simulink model "autopilota_v_22_last"  (R2020b)
settings: Solver=ode4  StartTime=0.0  StopTime=300  FixedStep=0.02  RelTol=1e-3
values from neighbouring files (symbols this model uses):
  alphavec_rad = deg2rad(alphavec)    [v2021_10_27_calcoloAerodinamica.m]
  attuatore_Amax = 20*(pi/180)    (= 0.349065850399)    [v2021_10_27_avvioSITL.m]    (also in v2021_10_27_calcoloAerodinamica.m)
  attuatore_Amin = -20*(pi/180)    (= -0.349065850399)    [v2021_10_27_avvioSITL.m]
  attuatore_Emax = 25*(pi/180)    (= 0.436332312999)    [v2021_10_27_avvioSITL.m]    (also in v2021_10_27_calcoloAerodinamica.m)
  attuatore_Emin = -25*(pi/180)    (= -0.436332312999)    [v2021_10_27_avvioSITL.m]
  attuatore_Rmax = 25*(pi/180)    (= 0.436332312999)    [v2021_10_27_avvioSITL.m]    (also in v2021_10_27_calcoloAerodinamica.m)
  attuatore_Rmin = -25*(pi/180)    (= -0.436332312999)    [v2021_10_27_avvioSITL.m]
  attuatore_Tmax = 0.99    [v2021_10_27_avvioSITL.m]
  attuatore_Tmin = 0    [v2021_10_27_avvioSITL.m]
  b = 2.62    [v2021_10_27_calcoloAerodinamica.m]
  betavec_rad = deg2rad(betavec)    [v2021_10_27_calcoloAerodinamica.m]
  bias = [baccxINI,baccyINI,bacczINI,bpINI,bqINI,brINI]    [v2021_10_27_avvioSITL.m]
  c = .32    (= 0.32)    [v2021_10_27_calcoloAerodinamica.m]
  cbar = .32    (= 0.32)    [v2021_10_27_calcoloAerodinamica.m]
  CD0 = 0.024    [v2021_10_27_calcoloAerodinamica.m]
  Clp = -0.5058    [v2021_10_27_calcoloAerodinamica.m]
  CLq = 19.166    [v2021_10_27_calcoloAerodinamica.m]
  Clr = 0.1459    [v2021_10_27_calcoloAerodinamica.m]
  Cmq = -81.796    [v2021_10_27_calcoloAerodinamica.m]
  Cnp = 0.007507    [v2021_10_27_calcoloAerodinamica.m]
  Cnr = -1.2593    [v2021_10_27_calcoloAerodinamica.m]
  CYp = 0.050728    [v2021_10_27_calcoloAerodinamica.m]
  CYr = 0.358925    [v2021_10_27_calcoloAerodinamica.m]
  deltaTtrim = 0.1    [v2021_10_27_avvioSITL.m]
  Dprop = 2*Rprop    (= 0.5334)    [v2021_10_27_calcoloAerodinamica.m]
  final_h = 35    [v2021_10_27_avvioSITL.m]
  g = [0 0 9.81]'    [v2021_10_27_calcoloAerodinamica.m]
  HINI = -State0.Pos0(3)    [v2021_10_27_avvioSITL.m]
  interventoA_05 = 20*0.8    (= 16)    [v2021_10_27_avvioSITL.m]
  interventoA_1 = 10    [v2021_10_27_avvioSITL.m]
  interventoE_05 = 25*0.8    (= 20)    [v2021_10_27_avvioSITL.m]
  interventoE_1 = 10    [v2021_10_27_avvioSITL.m]
  interventoT = 1*0.6    (= 0.6)    [v2021_10_27_avvioSITL.m]
  inv_A = 1    [v2021_10_27_avvioSITL.m]
  inv_comp_h = 1    [v2021_10_27_avvioSITL.m]
  inv_E = 1    [v2021_10_27_avvioSITL.m]
  inv_R = 1    [v2021_10_27_avvioSITL.m]
  inv_T = 1    [v2021_10_27_avvioSITL.m]
  Jeng = 0    [v2021_10_27_calcoloAerodinamica.m]
  Jprop = mprop*(Dprop^2)/12    (= 0.00422031414)    [v2021_10_27_calcoloAerodinamica.m]
  K_AW_B_AP_quota = 1000    [v2021_10_27_avvioSITL.m]
  K_AW_B_becc = -250    [v2021_10_27_avvioSITL.m]
  K_AW_B_imb = 0    [v2021_10_27_avvioSITL.m]
  K_AW_B_roll = 500    [v2021_10_27_avvioSITL.m]
  K_imb_inv = -0.001306    [v2021_10_27_avvioSITL.m]
  Kd_AP_rotta = 0.995    [v2021_10_27_avvioSITL.m]
  Kd_h_app = 0.085    [v2021_10_27_avvioSITL.m]
  Kd_h_flare = 0.01    [v2021_10_27_avvioSITL.m]
  Ki_AP_quota_select = 0.01936    [v2021_10_27_avvioSITL.m]
  Ki_AP_rotta = 0.002    [v2021_10_27_avvioSITL.m]
  Ki_AP_vel = 0.025175    [v2021_10_27_avvioSITL.m]
  Ki_becch = -0.1963    [v2021_10_27_avvioSITL.m]
  Ki_h_app = 0.055    [v2021_10_27_avvioSITL.m]
  Ki_h_cruise = 0.008    [v2021_10_27_avvioSITL.m]
  Ki_h_flare = 0.07    [v2021_10_27_avvioSITL.m]
  Ki_roll = 0.004528    [v2021_10_27_avvioSITL.m]
  Kp_AP_quota_hold_h = 0.5503    [v2021_10_27_avvioSITL.m]
  Kp_AP_quota_hold_l = 0.5503    [v2021_10_27_avvioSITL.m]
  Kp_AP_quota_select = 0.02647    [v2021_10_27_avvioSITL.m]
  Kp_AP_rotta = 0.520    (= 0.52)    [v2021_10_27_avvioSITL.m]
  Kp_AP_vel = 0.132175    [v2021_10_27_avvioSITL.m]
  Kp_becch = -0.30    (= -0.3)    [v2021_10_27_avvioSITL.m]
  Kp_comp_h = 0.035    [v2021_10_27_avvioSITL.m]
  Kp_h_app_max = 0.086    [v2021_10_27_avvioSITL.m]
  Kp_h_app_min = 0.01    [v2021_10_27_avvioSITL.m]
  Kp_h_cruise = 0.04    [v2021_10_27_avvioSITL.m]
  Kp_h_flare = 0.1    [v2021_10_27_avvioSITL.m]
  Kp_imb = 0.0019415    [v2021_10_27_avvioSITL.m]
  Kp_p = 0.006913    [v2021_10_27_avvioSITL.m]
  Kp_q = -0.025    [v2021_10_27_avvioSITL.m]
  Kp_roll = 0.0718    [v2021_10_27_avvioSITL.m]
  Kp_Rotta_ATO = 4    [v2021_10_27_avvioSITL.m]
  Kp_Rotta_psi = -0.01    [v2021_10_27_avvioSITL.m]
  latitudineINI = 41.854432*pi/180    (= 0.730497644952)    [v2021_10_27_avvioSITL.m]
  longitudineINI = 12.306650*pi/180    (= 0.214791562391)    [v2021_10_27_avvioSITL.m]
  matricepolinomi = [0.0816560564319 0.0869820125665 0.0279748858868 -4.51852057237 0.0146653626785 -0.925775006168 8.18052218957e-06 -1.47322908992e-05 7.59644694438e-06 0.00246695371279 9.02269223066e-06 0.000559334242525 ... (126 elements, 6x21)]    [coefficienti_curve_renard.mat]
  q = stato(11)    [measure_F1B.m]
  Q1B = [    2e-15;     2e-15 ... (first row only)    [COV_F1B.m]
  r = stato(12)    [measure_F1B.m]
  R1B = [     2e-14;             2e-14 ... (first row only)    [COV_F1B.m]
  rACtG = rACtP-rGP    [v2021_10_27_calcoloAerodinamica.m]
  rACwG = rACwP-rGP    [v2021_10_27_calcoloAerodinamica.m]
  rAHRSG = rAHRSP-rGP    [v2021_10_27_calcoloAerodinamica.m]
  rho = 1.21330    (= 1.2133)    [v2021_10_27_calcoloAerodinamica.m]
  rLEG = rLEP-rGP    [v2021_10_27_calcoloAerodinamica.m]
  rmglG = rmglP-rGP    [v2021_10_27_calcoloAerodinamica.m]
  rmgrG = rmgrP-rGP    [v2021_10_27_calcoloAerodinamica.m]
  rngG = rngP-rGP    [v2021_10_27_calcoloAerodinamica.m]
  rNPG = rNPP-rGP    [v2021_10_27_calcoloAerodinamica.m]
  rPG = -rGP    [v2021_10_27_calcoloAerodinamica.m]
  Rprop = 0.2667    [v2021_10_27_calcoloAerodinamica.m]
  S = b*cbar    (= 0.8384)    [v2021_10_27_calcoloAerodinamica.m]
  safe_phi = 55    [v2021_10_27_avvioSITL.m]
  safe_V = 40    [v2021_10_27_avvioSITL.m]
  Sensor_Offsets = [0,0,0]    [v2021_10_27_avvioSITL.m]
  T_cal = 0.4    [v2021_10_27_avvioSITL.m]
  theta_rot = 10    [v2021_10_27_avvioSITL.m]
  time_alarm_SAFE = 300    [v2021_10_27_avvioSITL.m]
  tsamp = 0.02    [v2021_10_27_avvioSITL.m]
  update = [2,2,2]    [v2021_10_27_avvioSITL.m]
  V_max = 35    [v2021_10_27_avvioSITL.m]
  V_stall = 15    [v2021_10_27_avvioSITL.m]
  vd_ini = 0    [v2021_10_27_avvioSITL.m]
  vel_wp1_al = 25    [v2021_10_27_avvioSITL.m]
  vel_wp2_al = 20    [v2021_10_27_avvioSITL.m]
  W = m*g    [v2021_10_27_calcoloAerodinamica.m]
  Zeng = rPG(3)    [v2021_10_27_calcoloAerodinamica.m]
undefined symbols (not defined in the file or in its folder): CldA, CLdE, CldR, CmdE, CndA, CndR, CYdA, CYdR, DiscIntNeverNeededParam, Earth, F, J_vec, MIL, Newton, Raphson, t_AP, WGS84
libraries: simulink_extras x38, pid_lib x9, simulink x5, dspsigops x4, aerolibwind2 x3, aerolibasang x2, aerolibtransform2sys x2, aerolibtransform2 x2, aerosimlib x1, shared6dof x1, aerolibatmos2 x1
(part 4 of 12)

== system autopilota_v_22_last/Subsystem1/Subsystem1/Subsystem ==
  modo : Inport
  rotta : Inport  Port=2
  velocita : Inport  Port=3
  quota : Inport  Port=4
  RC : Inport  Port=5
  heading : Inport  Port=6
  TAS : Inport  Port=7
  h : Inport  Port=8
  RC_default : Inport  Port=9
  <IAS> : Inport  Port=10
  <ALT> : Inport  Port=11
  <HDG> : Inport  Port=12
  <RC> : Inport  Port=13
  <Ingaggio_AP> : Inport  Port=14
  Enable : EnablePort
  Abs : Abs
  Data Type Conversion{,1..3} (4 alike) : DataTypeConversion  OutDataTypeStr=double
  Memory{,1..3,6} (5 alike) : Memory  InheritSampleTime=on
  Radians to Degrees3 : simulink_extras/Transformations/Radians to Degrees
  VETTORIALE : MATLAB Function  TreatAsAtomicUnit=on
  Out1 : Outport  VectorParamsAs1DForOutWhenUnconnected=off
  Out2 : Outport  Port=2  VectorParamsAs1DForOutWhenUnconnected=off
  Out3 : Outport  Port=3  VectorParamsAs1DForOutWhenUnconnected=off
  Out4 : Outport  Port=4  VectorParamsAs1DForOutWhenUnconnected=off
  wires:
  Data Type Conversion1/1 -> VETTORIALE/8(VELOCITA)
  Memory1/1 -> VETTORIALE/18(ALT_pre)
  VETTORIALE/5(ingaggio_AP_mem) -> Memory6/1
  Data Type Conversion2/1 -> VETTORIALE/9(QUOTA)
  VETTORIALE/8(ALT_pre_mem) -> Memory1/1
  Radians to Degrees3/1 -> VETTORIALE/11(HEADING)
  Memory6/1 -> VETTORIALE/15(ingaggio_AP_pre)
  h/1 -> VETTORIALE/13(h)
  Memory3/1 -> VETTORIALE/16(modo_pre)
  VETTORIALE/6(modo_pre_mem) -> Memory3/1
  Abs/1 -> VETTORIALE/10(RC)
  VETTORIALE/9(HDG_pre_mem) -> Memory/1
  Data Type Conversion3/1 -> Abs/1
  Memory/1 -> VETTORIALE/19(HDG_pre)
  Data Type Conversion/1 -> VETTORIALE/7(ROTTA)
  Memory2/1 -> VETTORIALE/17(IAS_pre)
  VETTORIALE/7(IAS_pre_mem) -> Memory2/1
  VETTORIALE/3(rotta_vett) -> Out3/1
  modo/1 -> VETTORIALE/1(modo)
  <ALT>/1 -> VETTORIALE/3(ALT)
  <RC>/1 -> VETTORIALE/5(I_RC)
  RC/1 -> Data Type Conversion3/1
  quota/1 -> Data Type Conversion2/1
  <Ingaggio_AP>/1 -> VETTORIALE/6(ingaggio_AP)
  TAS/1 -> VETTORIALE/12(TAS)
  heading/1 -> Radians to Degrees3/1
  velocita/1 -> Data Type Conversion1/1
  VETTORIALE/1(V_vett) -> Out1/1
  VETTORIALE/2(h_vett) -> Out2/1
  <IAS>/1 -> VETTORIALE/2(IAS)
  rotta/1 -> Data Type Conversion/1
  RC_default/1 -> VETTORIALE/14(RC_default)
  VETTORIALE/4(RC_vett) -> Out4/1
  <HDG>/1 -> VETTORIALE/4(HDG)

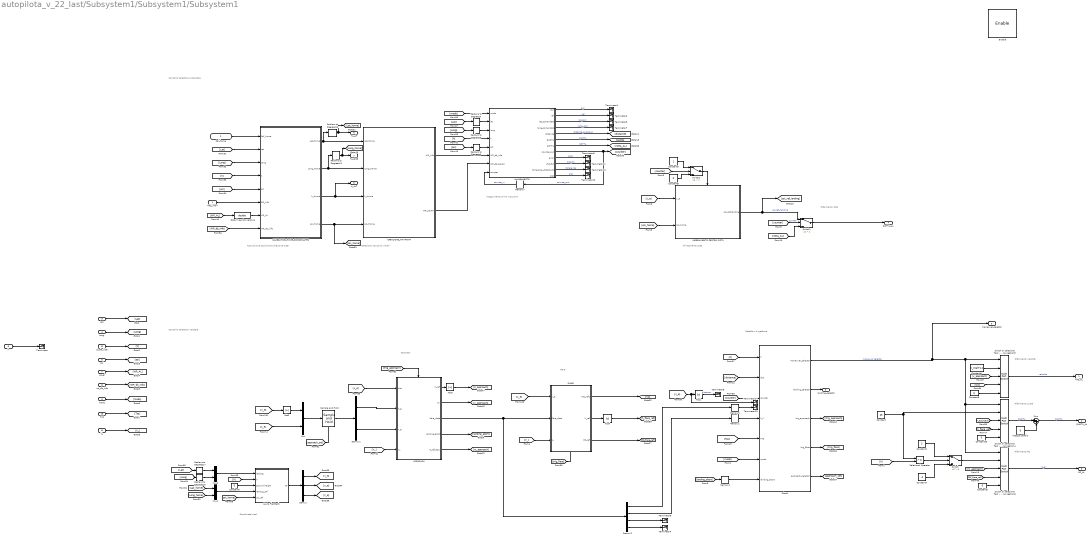
== system autopilota_v_22_last/Subsystem1/Subsystem1/Subsystem1 ==
  note: Approach
  note: Controllo traiettoria verticale
  note: Flare
  note: Coordinate locali
  note: Stateflow di gestione
  note: Controllo traiettoria orizzontale
  note: Acquisizione posizione
      | e direzione pista
  note: Creazione waypoint
      | virtuali
  note: Inseguimento primo
      | waypoint
  note: Allineamento
      | pista
  note: Riferimento rotta
  note: Riferimento velocità
  note: Riferimento quota
  note: Riferimento RC
  <GC_info> : Inport
  Cal_home : Inport  Port=2
  Lat : Inport  Port=3
  Long : Inport  Port=4
  h : Inport  Port=5
  psi : Inport  Port=6
  wp_al : Inport  Port=7
  wp_db_info : Inport  Port=8
  modo : Inport  Port=9
  TAS : Inport  Port=10
  V_ : Inport  Port=11
  quota_lidar : Inport  Port=12
  Enable : EnablePort
  ALLINEAMENTO : MATLAB Function  TreatAsAtomicUnit=on
  APPROACH : Subsystem
  Abs{1..4} (4 alike) : Abs
  CALIBRATING_HOME_COORDINATES : MATLAB Function  TreatAsAtomicUnit=on
  "CREAZIONE_WAYPOINT " : Subsystem
  Chart1 : Stateflow chart  TreatAsAtomicUnit=on
  Constant : Constant  Value=45
  Constant1 : Constant  Value=2  SampleTime=0.02
  Constant{5,8..10} (4 alike) : Constant  Value=0
  Constant3 : Constant
  Constant4 : Constant  Value=0  SampleTime=0.02
  Constant6 : Constant  Value=V_stall*1.4  SampleTime=0.02
  Constant7 : Constant  Value=-2  SampleTime=0.02
  Data Type Conversion4 : DataTypeConversion  OutDataTypeStr=double
  Demux : Demux  Outputs=3
  Demux1 : Demux  Outputs=2
  Demux2 : Demux
  FLARE : Subsystem
  INSEGUIMENTO CENTRO PISTA : Subsystem
  LLA to Flat Earth : Subsystem
  Memory1 : Memory
  Memory2 : Memory
  Memory5 : Memory
  Memory7 : Memory  InitialCondition=1  InheritSampleTime=on
  Mux : Mux  Inputs=2
  Mux1 : Mux  Inputs=2
  Mux2 : Mux  Inputs=2
  Radians to Degrees{4..6,10..11,16..17} (7 alike) : simulink_extras/Transformations/Radians to Degrees
  Relational Operator : RelationalOperator  OutDataTypeStr=boolean  RndMeth=Simplest
  Sample and Hold : dspsigops/Sample and Hold  trig=Rising edge  initCond=[0 0]  latchinput=off
  Sum : Sum  Inputs=|++
  Switch : Switch  Criteria=u2 > Threshold
  Switch di selezione Task - Waypoint navigation4 : MultiPortSwitch  Inputs=4
  Switch di selezione Task - Waypoint navigation5 : MultiPortSwitch  Inputs=4
  Switch di selezione Task - Waypoint navigation6 : MultiPortSwitch  Inputs=4
  Switch1 : Switch  Criteria=u2 > Threshold  Threshold=1
  Switch2 : Switch  Criteria=u2 > Threshold  Threshold=1
  Terminator{,1..5,7..14} (14 alike) : Terminator
  latezza carrello : Constant  Value=0
  TAS_AL : Outport  VectorParamsAs1DForOutWhenUnconnected=off
  QUOTA_AL : Outport  Port=2  VectorParamsAs1DForOutWhenUnconnected=off
  RC_AL : Outport  Port=3  VectorParamsAs1DForOutWhenUnconnected=off
  ROTTA_AL : Outport  Port=4  VectorParamsAs1DForOutWhenUnconnected=off
  landing_selector : Outport  Port=5  VectorParamsAs1DForOutWhenUnconnected=off
  H_LAT : Outport  Port=6  VectorParamsAs1DForOutWhenUnconnected=off
  H_LONG : Outport  Port=7  VectorParamsAs1DForOutWhenUnconnected=off
  H_ALT : Outport  Port=8  VectorParamsAs1DForOutWhenUnconnected=off
  maneuver_selector : Outport  Port=9
  wires:
  Chart1/1(maneuver_selector) -> maneuver_selector/1, Switch di selezione Task - Waypoint navigation6/1, Switch di selezione Task - Waypoint navigation4/1, Switch di selezione Task - Waypoint navigation5/1  "maneuver selector"
  LLA to Flat Earth/1(Xe) -> Demux/1
  Radians to Degrees11/1 -> H_LONG/1, [Long_home]
  Mux/1 -> Sample and Hold/1
  ALLINEAMENTO/4(long_comandato) -> Terminator7/1  "long_com"
  Mux1/1 -> LLA to Flat Earth/4(latlong_ref)
  [WP_db_info] -> CALIBRATING_HOME_COORDINATES/8(WP_db_info)
  Demux1/2 -> APPROACH/3(x_g)
  Abs2/1 -> Mux/1
  ALLINEAMENTO/3(lat_comandato) -> Terminator5/1  "lat_com"
  [rc_approach] -> Switch di selezione Task - Waypoint navigation6/3
  [V2] -> Switch di selezione Task - Waypoint navigation5/4
  [x_e] -> Terminator14/1, Abs1/1
  Abs4/1 -> [h_flare_ref]
  CALIBRATING_HOME_COORDINATES/3(h_Home) -> H_ALT/1, "CREAZIONE_WAYPOINT "/3(h_Home)
  [h] -> Chart1/1(h)
  [x_e] -> FLARE/1(x_e)
  [Long_home] -> Mux1/2
  APPROACH/3(flare_data) -> Demux2/1, FLARE/2(flare_data)
  CALIBRATING_HOME_COORDINATES/1(Lat_Home) -> Radians to Degrees10/1, "CREAZIONE_WAYPOINT "/1(Lat_Home)
  Demux/2 -> [y_e]
  FLARE/3(RC_ref) -> [RC_flare_ref]
  Chart1/4(trig_flare) -> [trig_flare]
  [h] -> LLA to Flat Earth/2(h)
  [Long] -> Radians to Degrees16/1
  Demux/3 -> [z_e]
  Demux2/2 -> Memory1/1
  Radians to Degrees10/1 -> H_LAT/1, [Lat_home]
  Sample and Hold/1 -> Demux1/1
  [trig_approach] -> APPROACH/Enable
  Switch/1 -> Switch di selezione Task - Waypoint navigation6/2
  Memory5/1 -> Terminator13/1
  Cal_home/1 -> CALIBRATING_HOME_COORDINATES/1(Cal_home)
  Demux2/3 -> Terminator3/1
  FLARE/2(h_ref) -> Abs4/1
  [z_e] -> Abs2/1
  [x_e] -> Mux/2
  CALIBRATING_HOME_COORDINATES/2(Long_Home) -> "CREAZIONE_WAYPOINT "/2(Long_Home), Radians to Degrees11/1
  Demux2/4 -> Terminator4/1
  FLARE/1(Tas_ref1) -> [V2]
  ALLINEAMENTO/7(ROTTA) -> [rotta_AL]  "ROTTA"
  APPROACH/2(V1) -> [v_approach]
  [V_] -> FLARE/3(V_)
  Chart1/5(approach_selector) -> [approach_sel]
  [h_approach] -> Switch di selezione Task - Waypoint navigation4/3
  [RC_flare_ref] -> Switch di selezione Task - Waypoint navigation6/4
  Chart1/3(trig_approach) -> [trig_approach]
  [Lat_home] -> Mux1/1
  ALLINEAMENTO/6(QUOTA) -> [quota]  "QUOTA"
  ALLINEAMENTO/8(counter_out) -> Memory7/1, [counter]  "counter_out"
  Demux/1 -> [x_e]
  Demux2/1 -> Memory5/1
  CALIBRATING_HOME_COORDINATES/4(psi_Home) -> [psi_home], "CREAZIONE_WAYPOINT "/4(psi_Home)
  Abs3/1 -> [h_approach]
  Mux2/1 -> LLA to Flat Earth/1(latlong)
  Chart1/2(landing_selector) -> landing_selector/1
  Constant/1 -> Switch di selezione Task - Waypoint navigation4/2, Relational Operator/1
  [h_flare_ref] -> Switch di selezione Task - Waypoint navigation4/4
  [v_approach] -> Switch di selezione Task - Waypoint navigation5/3
  [Tas] -> Chart1/5(TAS)
  APPROACH/1(h_ref) -> Abs3/1
  Data Type Conversion4/1 -> CALIBRATING_HOME_COORDINATES/7(WP_AL)
  [Lat] -> Radians to Degrees17/1
  Demux1/1 -> APPROACH/2(h_g)
  Constant4/1 -> LLA to Flat Earth/3(ground height)
  [psi] -> CALIBRATING_HOME_COORDINATES/5(psi)
  ALLINEAMENTO/2(vel) -> Terminator2/1  "vel"
  Radians to Degrees5/1 -> ALLINEAMENTO/3(long)
  [x_e] -> APPROACH/1(dist)
  Memory7/1 -> ALLINEAMENTO/8(counter)  "counter_in"
  [h] -> CALIBRATING_HOME_COORDINATES/4(h)
  [counter] -> Chart1/3(counter)
  Radians to Degrees4/1 -> ALLINEAMENTO/2(lat)
  [approach_sel] -> Sample and Hold/Trigger
  [Lat] -> Radians to Degrees4/1
  "CREAZIONE_WAYPOINT "/2(WP_param) -> ALLINEAMENTO/7(WP_db_param)
  [h] -> ALLINEAMENTO/4(h)
  [Long] -> Radians to Degrees5/1
  <GC_info>/1 -> CALIBRATING_HOME_COORDINATES/6(GC_info)
  ALLINEAMENTO/1(e_h) -> Terminator1/1  "e_h"
  Radians to Degrees6/1 -> ALLINEAMENTO/5(psi)
  Radians to Degrees16/1 -> Mux2/2
  [psi] -> Radians to Degrees6/1
  [WP_AL] -> Data Type Conversion4/1
  [modo] -> ALLINEAMENTO/1(modo)
  ALLINEAMENTO/5(distance) -> [distance]  "distance_autoland"
  Radians to Degrees17/1 -> Mux2/1
  "CREAZIONE_WAYPOINT "/1(WP_info) -> ALLINEAMENTO/6(WP_db_info)
  [trig_flare] -> FLARE/Enable
  Constant6/1 -> Switch di selezione Task - Waypoint navigation5/2
  [psi_home] -> LLA to Flat Earth/5(psi_ref)
  Sum/1 -> QUOTA_AL/1  "QUOTA"
  Switch di selezione Task - Waypoint navigation6/1 -> RC_AL/1  "rc_al"
  Switch di selezione Task - Waypoint navigation5/1 -> TAS_AL/1  "velocita"
  Lat/1 -> [Lat]
  Long/1 -> [Long]
  h/1 -> Terminator/1
  psi/1 -> [psi]
  wp_al/1 -> [WP_AL]
  wp_db_info/1 -> [WP_db_info]
  modo/1 -> [modo]
  TAS/1 -> [Tas]
  V_/1 -> [V_]
  Switch1/1 -> ROTTA_AL/1
  [h] -> Relational Operator/2
  Relational Operator/1 -> Switch/2
  Constant1/1 -> Switch/1
  Constant7/1 -> Switch/3
  [modo] -> Chart1/6(modo)
  APPROACH/4(landing_abort) -> [landing_abort]
  Memory1/1 -> Chart1/4(h_f)
  Memory2/1 -> Chart1/7(landing_abort)
  [landing_abort] -> Memory2/1
  [Lat] -> CALIBRATING_HOME_COORDINATES/2(Lat)
  [Long] -> CALIBRATING_HOME_COORDINATES/3(Long)
  [counter] -> Switch2/2
  [rotta_AL] -> Switch1/3
  [psi_home] -> INSEGUIMENTO CENTRO PISTA/2(psi_home)
  INSEGUIMENTO CENTRO PISTA/1(psi_ref_landing) -> [psi_ref_landing], Switch1/1  "psi_ref_landing"
  [y_e] -> INSEGUIMENTO CENTRO PISTA/1(y_e)
  [counter] -> Switch1/2  "counter"
  Constant8/1 -> Switch2/3
  Switch2/1 -> INSEGUIMENTO CENTRO PISTA/Enable
  Constant3/1 -> Switch2/1
  [V_] -> APPROACH/4(V_)
  APPROACH/5(rc_ref_app) -> [rc_approach]
  Switch di selezione Task - Waypoint navigation4/1 -> Sum/1  "QUOTA"
  latezza carrello/1 -> Sum/2
  quota_lidar/1 -> [h]
  Constant5/1 -> Switch di selezione Task - Waypoint navigation5/5
  Constant10/1 -> Switch di selezione Task - Waypoint navigation4/5
  Constant9/1 -> Switch di selezione Task - Waypoint navigation6/5
  ALLINEAMENTO/9(error) -> Terminator9/1  "error"
  ALLINEAMENTO/10(dist_fut) -> Terminator11/1  "dist_fut"
  ALLINEAMENTO/11(tolleranza_distWP_fut) -> Terminator10/1  "tolleranza"
  Abs1/1 -> Terminator8/1  "distance"
  [distance] -> Chart1/2(dist)
  ALLINEAMENTO/12(dist) -> Terminator12/1  "dist"

== system autopilota_v_22_last/Subsystem1/Subsystem1/Subsystem2 ==
  In1 : Inport
  In2 : Inport  Port=2
  In3 : Inport  Port=3
  In4 : Inport  Port=4
  In5 : Inport  Port=5
  In6 : Inport  Port=6
  <GC_info> : Inport  Port=7
  Enable : EnablePort
  Memory4 : Memory  InitialCondition=1  InheritSampleTime=on
  Radians to Degrees : simulink_extras/Transformations/Radians to Degrees
  Radians to Degrees1 : simulink_extras/Transformations/Radians to Degrees
  Radians to Degrees2 : simulink_extras/Transformations/Radians to Degrees
  Terminator : Terminator
  Terminator1 : Terminator
  Terminator2 : Terminator
  WAYPOINTS : MATLAB Function  TreatAsAtomicUnit=on
  WAYPOINTS2 : MATLAB Function  Commented=on  TreatAsAtomicUnit=on
  WAYPOINTS3 : MATLAB Function  Commented=on  TreatAsAtomicUnit=on
  saturatore V : Saturate  UpperLimit=40  LowerLimit=15
  saturatore V1 : Saturate  UpperLimit=2  LowerLimit=-2
  RC : Outport  VectorParamsAs1DForOutWhenUnconnected=off
  VELOCITA : Outport  Port=2  VectorParamsAs1DForOutWhenUnconnected=off
  Out3 : Outport  Port=3  VectorParamsAs1DForOutWhenUnconnected=off
  Out4 : Outport  Port=4  VectorParamsAs1DForOutWhenUnconnected=off
  wires:
  WAYPOINTS/8(counter_out) -> Memory4/1
  saturatore V1/1 -> RC/1  "RC"
  Radians to Degrees1/1 -> WAYPOINTS/2(long)
  WAYPOINTS/4(long_comandato) -> Terminator1/1
  Radians to Degrees/1 -> WAYPOINTS/1(lat)
  WAYPOINTS/2(vel) -> saturatore V/1
  WAYPOINTS/1(e_h) -> saturatore V1/1
  WAYPOINTS/5(distance) -> Terminator2/1
  WAYPOINTS/3(lat_comandato) -> Terminator/1
  Radians to Degrees2/1 -> WAYPOINTS/4(psi)
  Memory4/1 -> WAYPOINTS/8(counter)
  In1/1 -> Radians to Degrees/1
  In3/1 -> WAYPOINTS/3(h)
  In4/1 -> Radians to Degrees2/1
  In2/1 -> Radians to Degrees1/1
  WAYPOINTS/7(ROTTA) -> Out4/1
  In5/1 -> WAYPOINTS/5(WP_db_info)
  In6/1 -> WAYPOINTS/6(WP_db_param)
  <GC_info>/1 -> WAYPOINTS/7(GC_info)
  saturatore V/1 -> VELOCITA/1  "VELOCITA"
  WAYPOINTS/6(QUOTA) -> Out3/1

== system autopilota_v_22_last/Subsystem1/Subsystem1/Subsystem3 ==
  In1 : Inport
  In2 : Inport  Port=2
  In3 : Inport  Port=3
  In4 : Inport  Port=4
  In5 : Inport  Port=5
  In6 : Inport  Port=6
  In7 : Inport  Port=7
  In8 : Inport  Port=8
  Enable : EnablePort
  GO_HOME : MATLAB Function  TreatAsAtomicUnit=on
  Radians to Degrees12 : simulink_extras/Transformations/Radians to Degrees
  Radians to Degrees13 : simulink_extras/Transformations/Radians to Degrees
  Radians to Degrees9 : simulink_extras/Transformations/Radians to Degrees
  Out1 : Outport  VectorParamsAs1DForOutWhenUnconnected=off
  Out2 : Outport  Port=2  VectorParamsAs1DForOutWhenUnconnected=off
  Out3 : Outport  Port=3  VectorParamsAs1DForOutWhenUnconnected=off
  Out4 : Outport  Port=4  VectorParamsAs1DForOutWhenUnconnected=off
  wires:
  GO_HOME/1(V_goHome) -> Out1/1
  GO_HOME/4(rotta_goHome) -> Out4/1
  GO_HOME/3(RC_goHome) -> Out3/1
  Radians to Degrees9/1 -> GO_HOME/4(psi)
  Radians to Degrees12/1 -> GO_HOME/1(lat)
  In2/1 -> Radians to Degrees13/1
  Radians to Degrees13/1 -> GO_HOME/2(long)
  In3/1 -> GO_HOME/3(h)
  In4/1 -> Radians to Degrees9/1
  In6/1 -> GO_HOME/6(Long_Home)
  In8/1 -> GO_HOME/8(V_goHome_rif)
  In5/1 -> GO_HOME/5(Lat_Home)
  In1/1 -> Radians to Degrees12/1
  GO_HOME/2(h_goHome) -> Out2/1
  In7/1 -> GO_HOME/7(h_goHome_rif)

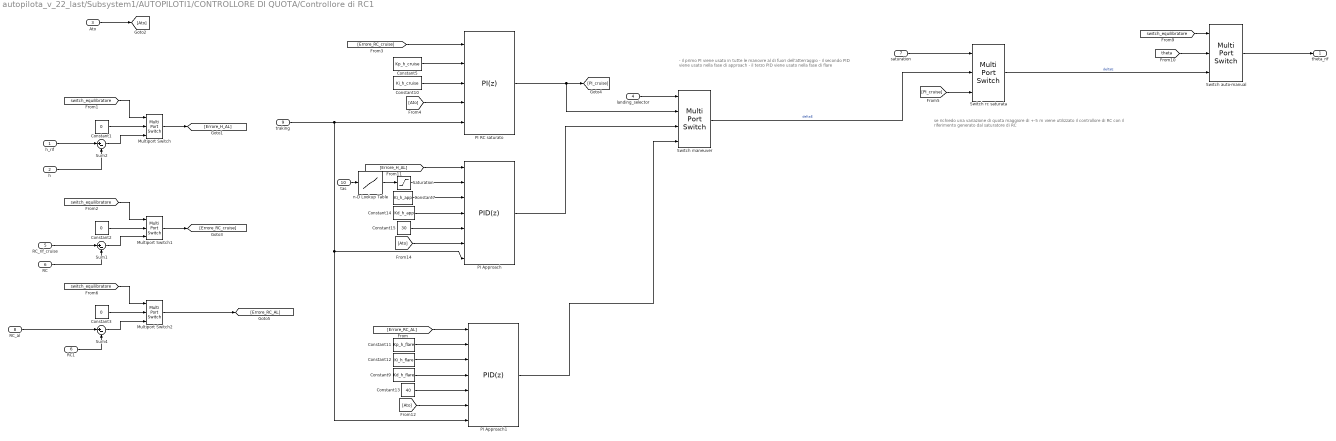
== system autopilota_v_22_last/Subsystem1/AUTOPILOTI1/CONTROLLORE DI QUOTA/Controllore di RC1 ==
  note: - il primo PI viene usato in tutte le manovre al di fuori dell'atterraggio
      | - il secondo PID viene usato nella fase di approach
      | - il terzo PID viene usato nella fase di flare
  note: se richiedo una variazione di quota maggiore di +-5 m viene utilizzato il controllore di RC
      | con il riferimento generato dal saturatore di RC
  h_rif : Inport
  h : Inport  Port=2
  "Ato " : Inport  Port=3
  landing_selector : Inport  Port=4
  RC_rif_cruise : Inport  Port=5
  RC : Inport  Port=6
  saturation : Inport  Port=7
  "RC_al " : Inport  Port=8
  traking : Inport  Port=9
  tas : Inport  Port=10
  Constant1 : Constant  Value=0  SampleTime=t_AP
  Constant10 : Constant  Value=Ki_h_cruise  SampleTime=t_AP
  Constant11 : Constant  Value=Kp_h_flare  SampleTime=0.02
  Constant12 : Constant  Value=Ki_h_flare  SampleTime=0.02
  Constant13 : Constant  Value=40  SampleTime=0.02
  Constant14 : Constant  Value=Kd_h_app  SampleTime=0.02
  Constant15 : Constant  Value=30  SampleTime=0.02
  Constant2 : Constant  Value=0  SampleTime=t_AP
  Constant3 : Constant  Value=0  SampleTime=t_AP
  Constant5 : Constant  Value=Kp_h_cruise  SampleTime=t_AP
  Constant7 : Constant  Value=Ki_h_app  SampleTime=0.02
  Constant9 : Constant  Value=Kd_h_flare  SampleTime=0.02
  Multiport Switch : MultiPortSwitch  DataPortOrder=Zero-based contiguous  Inputs=2  zeroidx=on
  Multiport Switch1 : MultiPortSwitch  DataPortOrder=Zero-based contiguous  Inputs=2  zeroidx=on
  Multiport Switch2 : MultiPortSwitch  DataPortOrder=Zero-based contiguous  Inputs=2  zeroidx=on
  PI Approach : pid_lib/PID Controller  Controller=PID  Form=Parallel  TimeDomain=Discrete-time  UseExternalTs=off  SampleTime=0.02  IntegratorMethod=Forward Euler  FilterMethod=Forward Euler  ControllerParametersSource=external  P=1  I=1  D=0  UseFilter=on  N=100  TunerSelectOption=Transfer Function Based (PID Tuner App)  InitialConditionSource=internal  InitialConditionForIntegrator=0  InitialConditionForFilter=0  DifferentiatorICPrevScaledInput=0  ExternalReset=rising  TrackingMode=on  Kt=1  LimitOutput=off  SatLimitsSource=internal  UpperSaturationLimit=0.7  LowerSaturationLimit=-0.7  LinearizeAsGain=off  AntiWindupMode=back-calculation  Kb=1  POutMin=[]  POutMax=[]  IOutMin=[]  IOutMax=[]  DOutMin=[]  DOutMax=[]  NOutMin=[]  NOutMax=[]  SumOutMin=[]  SumOutMax=[]  SaturationOutMin=[]  SaturationOutMax=[]  PParamMin=[]  PParamMax=[]  IParamMin=[]  IParamMax=[]  DParamMin=[]  DParamMax=[]  NParamMin=[]  NParamMax=[]  KbParamMin=[]  KbParamMax=[]  KtParamMin=[]  KtParamMax=[]  KbOutMin=[]  KbOutMax=[]  KtOutMin=[]  KtOutMax=[]  IntegratorOutMin=[]  IntegratorOutMax=[]  FilterOutMin=[]  FilterOutMax=[]  SumI1OutMin=[]  SumI1OutMax=[]  SumI2OutMin=[]  SumI2OutMax=[]  SumI3OutMin=[]  SumI3OutMax=[]  SumI4OutMin=[]  SumI4OutMax=[]  SumDOutMin=[]  SumDOutMax=[]  DifferentiatorOutMin=[]  DifferentiatorOutMax=[]  FilterDiffOutCoefMin=[]  FilterDiffOutCoefMax=[]  ReciprocalOutMin=[]  ReciprocalOutMax=[]  SumDenOutMin=[]  SumDenOutMax=[]  SumNumOutMin=[]  SumNumOutMax=[]  DivideOutMin=[]  DivideOutMax=[]  UdiffTsProdOutMin=[]  UdiffTsProdOutMax=[]  NTsProdOutMin=[]  NTsProdOutMax=[]  UintegralTsProdOutMin=[]  UintegralTsProdOutMax=[]  UngainTsProdOutMin=[]  UngainTsProdOutMax=[]  IntegratorContinuousStateAttributes=''  IntegratorStateMustResolveToSignalObject=off  IntegratorRTWStateStorageClass=Auto  FilterContinuousStateAttributes=''  FilterStateMustResolveToSignalObject=off  FilterRTWStateStorageClass=Auto  ParallelPVariant=ExternalParameters  IdealPVariant=Disabled  IVariant=ExternalParameters  DVariant=ExternalParameters  IntegratorVariant=Discrete  SatVariant=Disabled  AWVariant=Passthrough  PCopyVariant=Disabled  TRVariant=Enabled  FdbkBlocksVariant=Forward  IdealPFdbkVariant=Disabled  SatFdbkVariant=Disabled  DerivativeFilterVariant=ForwardEulerFilter  NVariant=ExternalParameters  NCopyVariant=Disabled  FilterICVariant=InternalICsFilter  IntegratorICVariant=InternalICs  ExternalResetVariant=ExternalReset  TRSumVariant=TrackingMode  SumFdbkVariant=Disabled  SumVariant=Sum_PID  TsampFilterVariant=InternalTs  TsampNgainVariant=Passthrough  TsampIntegralVariant=Passthrough  ExternalSaturationOutDataTypeStr=Inherit: Same as second input
  PI Approach1 : pid_lib/PID Controller  Controller=PID  Form=Parallel  TimeDomain=Discrete-time  UseExternalTs=off  SampleTime=0.02  IntegratorMethod=Forward Euler  FilterMethod=Forward Euler  ControllerParametersSource=external  P=1  I=1  D=0  UseFilter=on  N=100  TunerSelectOption=Transfer Function Based (PID Tuner App)  InitialConditionSource=internal  InitialConditionForIntegrator=0  InitialConditionForFilter=0  DifferentiatorICPrevScaledInput=0  ExternalReset=rising  TrackingMode=on  Kt=1  LimitOutput=off  SatLimitsSource=internal  UpperSaturationLimit=0.7  LowerSaturationLimit=-0.7  LinearizeAsGain=off  AntiWindupMode=back-calculation  Kb=1  POutMin=[]  POutMax=[]  IOutMin=[]  IOutMax=[]  DOutMin=[]  DOutMax=[]  NOutMin=[]  NOutMax=[]  SumOutMin=[]  SumOutMax=[]  SaturationOutMin=[]  SaturationOutMax=[]  PParamMin=[]  PParamMax=[]  IParamMin=[]  IParamMax=[]  DParamMin=[]  DParamMax=[]  NParamMin=[]  NParamMax=[]  KbParamMin=[]  KbParamMax=[]  KtParamMin=[]  KtParamMax=[]  KbOutMin=[]  KbOutMax=[]  KtOutMin=[]  KtOutMax=[]  IntegratorOutMin=[]  IntegratorOutMax=[]  FilterOutMin=[]  FilterOutMax=[]  SumI1OutMin=[]  SumI1OutMax=[]  SumI2OutMin=[]  SumI2OutMax=[]  SumI3OutMin=[]  SumI3OutMax=[]  SumI4OutMin=[]  SumI4OutMax=[]  SumDOutMin=[]  SumDOutMax=[]  DifferentiatorOutMin=[]  DifferentiatorOutMax=[]  FilterDiffOutCoefMin=[]  FilterDiffOutCoefMax=[]  ReciprocalOutMin=[]  ReciprocalOutMax=[]  SumDenOutMin=[]  SumDenOutMax=[]  SumNumOutMin=[]  SumNumOutMax=[]  DivideOutMin=[]  DivideOutMax=[]  UdiffTsProdOutMin=[]  UdiffTsProdOutMax=[]  NTsProdOutMin=[]  NTsProdOutMax=[]  UintegralTsProdOutMin=[]  UintegralTsProdOutMax=[]  UngainTsProdOutMin=[]  UngainTsProdOutMax=[]  IntegratorContinuousStateAttributes=''  IntegratorStateMustResolveToSignalObject=off  IntegratorRTWStateStorageClass=Auto  FilterContinuousStateAttributes=''  FilterStateMustResolveToSignalObject=off  FilterRTWStateStorageClass=Auto  ParallelPVariant=ExternalParameters  IdealPVariant=Disabled  IVariant=ExternalParameters  DVariant=ExternalParameters  IntegratorVariant=Discrete  SatVariant=Disabled  AWVariant=Passthrough  PCopyVariant=Disabled  TRVariant=Enabled  FdbkBlocksVariant=Forward  IdealPFdbkVariant=Disabled  SatFdbkVariant=Disabled  DerivativeFilterVariant=ForwardEulerFilter  NVariant=ExternalParameters  NCopyVariant=Disabled  FilterICVariant=InternalICsFilter  IntegratorICVariant=InternalICs  ExternalResetVariant=ExternalReset  TRSumVariant=TrackingMode  SumFdbkVariant=Disabled  SumVariant=Sum_PID  TsampFilterVariant=InternalTs  TsampNgainVariant=Passthrough  TsampIntegralVariant=Passthrough  ExternalSaturationOutDataTypeStr=Inherit: Same as second input
  PI RC saturato : pid_lib/PID Controller  Controller=PI  Form=Parallel  TimeDomain=Discrete-time  UseExternalTs=off  SampleTime=0.02  IntegratorMethod=Forward Euler  FilterMethod=Forward Euler  ControllerParametersSource=external  P=1  I=1  D=0  UseFilter=on  N=100  TunerSelectOption=Transfer Function Based (PID Tuner App)  InitialConditionSource=internal  InitialConditionForIntegrator=0  InitialConditionForFilter=0  DifferentiatorICPrevScaledInput=0  ExternalReset=rising  TrackingMode=on  Kt=1  LimitOutput=off  SatLimitsSource=internal  UpperSaturationLimit=0.7  LowerSaturationLimit=-0.7  LinearizeAsGain=off  AntiWindupMode=back-calculation  Kb=1  POutMin=[]  POutMax=[]  IOutMin=[]  IOutMax=[]  DOutMin=[]  DOutMax=[]  NOutMin=[]  NOutMax=[]  SumOutMin=[]  SumOutMax=[]  SaturationOutMin=[]  SaturationOutMax=[]  PParamMin=[]  PParamMax=[]  IParamMin=[]  IParamMax=[]  DParamMin=[]  DParamMax=[]  NParamMin=[]  NParamMax=[]  KbParamMin=[]  KbParamMax=[]  KtParamMin=[]  KtParamMax=[]  KbOutMin=[]  KbOutMax=[]  KtOutMin=[]  KtOutMax=[]  IntegratorOutMin=[]  IntegratorOutMax=[]  FilterOutMin=[]  FilterOutMax=[]  SumI1OutMin=[]  SumI1OutMax=[]  SumI2OutMin=[]  SumI2OutMax=[]  SumI3OutMin=[]  SumI3OutMax=[]  SumI4OutMin=[]  SumI4OutMax=[]  SumDOutMin=[]  SumDOutMax=[]  DifferentiatorOutMin=[]  DifferentiatorOutMax=[]  FilterDiffOutCoefMin=[]  FilterDiffOutCoefMax=[]  ReciprocalOutMin=[]  ReciprocalOutMax=[]  SumDenOutMin=[]  SumDenOutMax=[]  SumNumOutMin=[]  SumNumOutMax=[]  DivideOutMin=[]  DivideOutMax=[]  UdiffTsProdOutMin=[]  UdiffTsProdOutMax=[]  NTsProdOutMin=[]  NTsProdOutMax=[]  UintegralTsProdOutMin=[]  UintegralTsProdOutMax=[]  UngainTsProdOutMin=[]  UngainTsProdOutMax=[]  IntegratorContinuousStateAttributes=''  IntegratorStateMustResolveToSignalObject=off  IntegratorRTWStateStorageClass=Auto  FilterContinuousStateAttributes=''  FilterStateMustResolveToSignalObject=off  FilterRTWStateStorageClass=Auto  ParallelPVariant=ExternalParameters  IdealPVariant=Disabled  IVariant=ExternalParameters  DVariant=Disabled  IntegratorVariant=Discrete  SatVariant=Disabled  AWVariant=Passthrough  PCopyVariant=Disabled  TRVariant=Enabled  FdbkBlocksVariant=Forward  IdealPFdbkVariant=Disabled  SatFdbkVariant=Disabled  DerivativeFilterVariant=Disabled  NVariant=Disabled  NCopyVariant=Disabled_SignalSpec  FilterICVariant=Disabled  IntegratorICVariant=InternalICs  ExternalResetVariant=ExternalReset  TRSumVariant=TrackingMode  SumFdbkVariant=Disabled  SumVariant=Sum_PI  TsampFilterVariant=InternalTs  TsampNgainVariant=Passthrough  TsampIntegralVariant=Passthrough  ExternalSaturationOutDataTypeStr=Inherit: Same as second input
  RC1 : InportShadow  Port=6
  Saturation : Saturate  UpperLimit=0.046  LowerLimit=0.01
  Sum1 : Sum  Inputs=|+-
  Sum2 : Sum  Inputs=|+-
  Sum4 : Sum  Inputs=|+-
  Switch auto-manual : MultiPortSwitch  DataPortOrder=Zero-based contiguous  Inputs=2  zeroidx=on
  Switch maneuver : MultiPortSwitch  DataPortOrder=Zero-based contiguous  zeroidx=on
  Switch rc saturata : MultiPortSwitch  DataPortOrder=Zero-based contiguous  Inputs=2  zeroidx=on
  n-D Lookup Table : Lookup_n-D  NumberOfTableDimensions=1  BreakpointsForDimension1="[V_stall*1.2  V_max*0.75]"  Table=[Kp_h_app_max Kp_h_app_min]  RndMeth=Simplest  InputSameDT=on
  theta_rif : Outport  VectorParamsAs1DForOutWhenUnconnected=off
  wires:
  landing_selector/1 -> Switch maneuver/1
  [Ato] -> PI Approach/6
  "Ato "/1 -> [Ato]
  [Errore_H_AL] -> PI Approach/1
  [switch_equilibratore] -> Switch auto-manual/1
  [theta] -> Switch auto-manual/2
  Multiport Switch/1 -> [Errore_H_AL]
  [switch_equilibratore] -> Multiport Switch/1
  Constant1/1 -> Multiport Switch/2
  Sum2/1 -> Multiport Switch/3
  h/1 -> Sum2/2
  h_rif/1 -> Sum2/1
  Saturation/1 -> PI Approach/2
  Constant7/1 -> PI Approach/3
  RC_rif_cruise/1 -> Sum1/1
  Sum1/1 -> Multiport Switch1/3
  Constant2/1 -> Multiport Switch1/2
  Multiport Switch1/1 -> [Errore_RC_cruise]
  [switch_equilibratore] -> Multiport Switch1/1
  Switch maneuver/1 -> Switch rc saturata/2  "deltaE"
  RC/1 -> Sum1/2
  saturation/1 -> Switch rc saturata/1
  Switch rc saturata/1 -> Switch auto-manual/3  "deltaE"
  PI RC saturato/1 -> [PI_cruise], Switch maneuver/2
  Constant5/1 -> PI RC saturato/2
  [Ato] -> PI RC saturato/4
  Constant10/1 -> PI RC saturato/3
  [Errore_RC_cruise] -> PI RC saturato/1
  [PI_cruise] -> Switch rc saturata/3
  "RC_al "/1 -> Sum4/1
  [switch_equilibratore] -> Multiport Switch2/1
  RC1/1 -> Sum4/2
  Multiport Switch2/1 -> [Errore_RC_AL]
  Constant3/1 -> Multiport Switch2/2
  Sum4/1 -> Multiport Switch2/3
  PI Approach/1 -> Switch maneuver/3
  [Errore_RC_AL] -> PI Approach1/1
  Constant11/1 -> PI Approach1/2
  Constant12/1 -> PI Approach1/3
  [Ato] -> PI Approach1/6
  Switch auto-manual/1 -> theta_rif/1
  PI Approach1/1 -> Switch maneuver/4
  traking/1 -> PI Approach1/7, PI Approach/7, PI RC saturato/5
  Constant9/1 -> PI Approach1/4
  Constant13/1 -> PI Approach1/5
  Constant14/1 -> PI Approach/4
  Constant15/1 -> PI Approach/5
  tas/1 -> n-D Lookup Table/1
  n-D Lookup Table/1 -> Saturation/1

== system autopilota_v_22_last/Subsystem1/AUTOPILOTI1/CONTROLLORE DI QUOTA/Saturazione RC  ==
  V : Inport
  RC : Inport  Port=2
  Constant : Constant  Value=-5  SampleTime=t_AP
  Lookup Table2 : Lookup  InputValues=[15;20;25;30;35;40]  Table=[2;2.5;3;3.5;4;4]
  Saturation Dynamic1 : simulink/Discontinuities/Saturation Dynamic  OutMin=[]  OutMax=[]  OutDataTypeStr=Inherit: Same as second input  OutDataType=fixdt(1, 16)  OutScaling=2^-10  DoSatur=off
  RC_verficata : Outport  VectorParamsAs1DForOutWhenUnconnected=off
  wires:
  V/1 -> Lookup Table2/1
  RC/1 -> Saturation Dynamic1/2
  Lookup Table2/1 -> Saturation Dynamic1/1
  Constant/1 -> Saturation Dynamic1/3
  Saturation Dynamic1/1 -> RC_verficata/1

== system autopilota_v_22_last/Subsystem1/AUTOPILOTI1/CONTROLLORE DI ROTTA/ATO ==
  In1 : Inport
  In2 : Inport  Port=2
  In3 : Inport  Port=3
  In4 : Inport  Port=4
  Constant3 : Constant  Value=Kp_Rotta_ATO
  Constant4 : Constant  Value=0
  Multiport Switch2 : MultiPortSwitch  DataPortOrder=Zero-based contiguous  Inputs=2  zeroidx=on
  Multiport Switch3 : MultiPortSwitch  DataPortOrder=Zero-based contiguous  Inputs=2  zeroidx=on
  Switch3 : Switch  Criteria=u2 > Threshold  Threshold=2
  Switch4 : Switch  Criteria=u2 > Threshold  Threshold=2
  Out1 : Outport  VectorParamsAs1DForOutWhenUnconnected=off
  "Out2 " : Outport  Port=2  VectorParamsAs1DForOutWhenUnconnected=off
  wires:
  Switch3/1 -> Out1/1
  Constant4/1 -> Multiport Switch3/3
  In1/1 -> Switch3/1, Multiport Switch2/2
  [Switch_ATO] -> Multiport Switch3/1
  [Alt] -> Switch3/2
  Multiport Switch2/1 -> Switch3/3
  [Alt] -> Switch4/2
  [Switch_ATO] -> Multiport Switch2/1
  In4/1 -> Switch4/1, Multiport Switch3/2
  Constant3/1 -> Multiport Switch2/3
  Switch4/1 -> "Out2 "/1
  In2/1 -> [Switch_ATO]
  In3/1 -> [Alt]
  Multiport Switch3/1 -> Switch4/3

== system autopilota_v_22_last/Subsystem1/AUTOPILOTI1/CONTROLLORE DI ROTTA/calcolo errore Psi  ==
  psi_ref (°) : Inport
  psi (rad) : Inport  Port=2
  Constant : Constant  Value=360  SampleTime=t_AP
  Constant1 : Constant  Value=360  SampleTime=t_AP
  Constant2 : Constant  Value=360  SampleTime=t_AP
  Degrees to Radians : simulink_extras/Transformations/Degrees to Radians
  Math Function : Math  Operator=mod  SignedPower=on  SaturateOnIntegerOverflow=on
  Radians to Degrees : simulink_extras/Transformations/Radians to Degrees
  Sum : Sum  Inputs=|+-
  Sum1 : Sum  Inputs=|+-
  Sum2 : Sum  Inputs=|++
  Switch : Switch  Threshold=180
  Switch1 : Switch  Threshold=-180
  psi_err : Outport  VectorParamsAs1DForOutWhenUnconnected=off
  wires:
  Radians to Degrees/1 -> Math Function/1
  Degrees to Radians/1 -> psi_err/1
  Switch1/1 -> Degrees to Radians/1
  Sum2/1 -> Switch1/3
  Constant2/1 -> Sum2/2
  Switch/1 -> Switch1/1
  Sum/1 -> Sum2/1, Switch1/2, Switch/3, Switch/2, Sum1/1
  Constant1/1 -> Sum1/2
  Sum1/1 -> Switch/1
  Math Function/1 -> Sum/2
  Constant/1 -> Math Function/2
  psi (rad)/1 -> Radians to Degrees/1
  psi_ref (°)/1 -> Sum/1

== system autopilota_v_22_last/Subsystem1/AUTOPILOTI1/CONTROLLORE DI VELOCITA'/throttle - landing ==
  AL : Inport
  In2 : Inport  Port=2
  Alt : Inport  Port=3
  In4 : Inport  Port=4
  Constant : Constant  Value=4
  Constant1 : Constant  Value=0
  Constant3 : Constant  Value=0
  Enabled Subsystem : Subsystem  TreatAsAtomicUnit=on
  Hit Crossing : HitCross  HitCrossingOffset=0.3  HitCrossingDirection=falling
  Sum : Sum  Inputs=+-
  Switch : Switch  Criteria=u2 > Threshold
  Switch1 : Switch  Criteria=u2 ~= 0
  throttle - landing : MultiPortSwitch  DataPortOrder=Zero-based contiguous  Inputs=2  zeroidx=on
  Out1 : Outport  VectorParamsAs1DForOutWhenUnconnected=off
  wires:
  Switch/1 -> throttle - landing/3
  throttle - landing/1 -> Switch1/1
  AL/1 -> throttle - landing/1
  Alt/1 -> Hit Crossing/1
  In2/1 -> Switch/1, throttle - landing/2
  Constant3/1 -> Switch/3
  Hit Crossing/1 -> Enabled Subsystem/Trigger
  Enabled Subsystem/1(Out1) -> Switch/2
  In4/1 -> Sum/1
  Constant/1 -> Sum/2
  Sum/1 -> Switch1/2
  Switch1/1 -> Out1/1
  Constant1/1 -> Switch1/3

== system autopilota_v_22_last/Subsystem1/CONTROLLI INTERNI E SWITCH1/AENEA II_SITL1/Forze aerodinamiche ==
  ωb : Inport
  qbar : Inport  Port=2
  Vect_Comandi : Inport  Port=3
  Vect_Costanti : Inport  Port=4
  "Vbpolare " : Inport  Port=5
  Bus Creator : BusCreator  Inputs=3
  Bus Selector : BusSelector  OutputSignals=α,β
  Bus Selector1 : BusSelector  OutputSignals=Coef_Geometrici.S
  Demux : Demux  Outputs=3
  Forze assi vento/q : Subsystem
  MATLAB Function : MATLAB Function  TreatAsAtomicUnit=on
  Matrix Multiply : Product  Multiplication=Matrix(*)
  Momenti /press din : Subsystem
  Product : Product  Inputs=3
  Product2 : Product
  FA_B : Outport  VectorParamsAs1DForOutWhenUnconnected=off
  MA_B : Outport  Port=2  VectorParamsAs1DForOutWhenUnconnected=off
  CL : Outport  Port=3  VectorParamsAs1DForOutWhenUnconnected=off
  wires:
  Product2/1 -> MA_B/1
  Product/1 -> FA_B/1
  qbar/1 -> Product/3, Product2/1
  ωb/1 -> Demux/1
  Demux/1 -> Bus Creator/1  "p"
  Demux/2 -> Bus Creator/2  "q"
  Demux/3 -> Bus Creator/3  "r"
  Bus Selector/1 -> MATLAB Function/1(alpha)  "<α>"
  Bus Selector/2 -> MATLAB Function/2(beta)  "<β>"
  MATLAB Function/1(Lbw) -> Matrix Multiply/1
  Matrix Multiply/1 -> Product/2  "FA_B/q"
  Momenti /press din/1(MA_B/q) -> Product2/2
  Forze assi vento/q/1(FA_W/q) -> Matrix Multiply/2
  Vect_Comandi/1 -> Forze assi vento/q/1(Vect_Comandi), Momenti /press din/1(Vect_Comandi)
  "Vbpolare "/1 -> Bus Selector/1, Forze assi vento/q/3("Vbpolare "), Momenti /press din/3("Vbpolare ")
  Bus Creator/1 -> Momenti /press din/4(ωb), Forze assi vento/q/4(ωb)  "ωb"
  Vect_Costanti/1 -> Bus Selector1/1, Forze assi vento/q/2(Vect_Costanti), Momenti /press din/2(Vect_Costanti)
  Bus Selector1/1 -> Product/1  "<S>"
  Forze assi vento/q/2(CL) -> CL/1

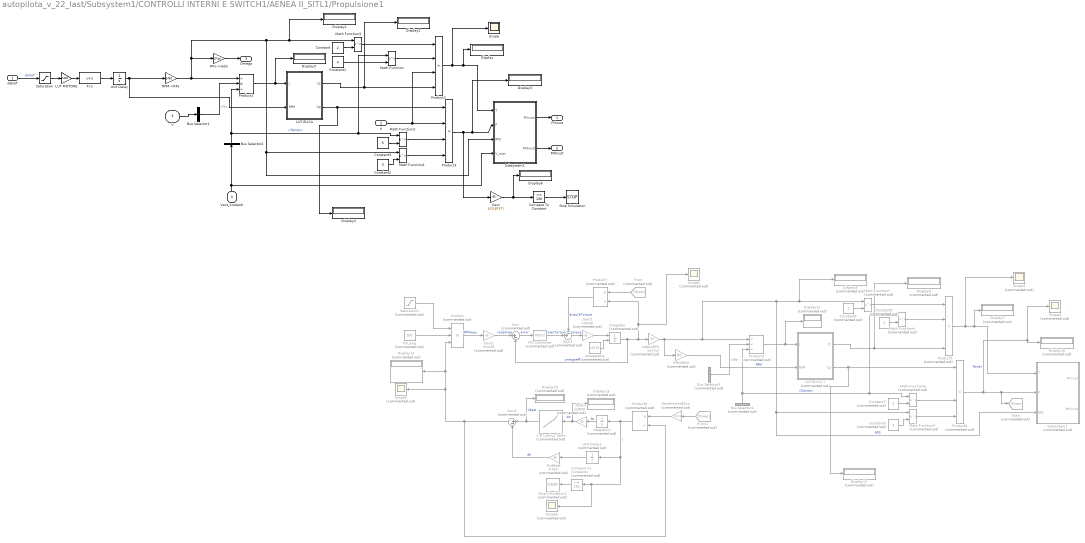
== system autopilota_v_22_last/Subsystem1/CONTROLLI INTERNI E SWITCH1/AENEA II_SITL1/Propulsione1 ==
  "deltaT " : Inport
  ρ : Inport  Port=2
  V : Inport  Port=3
  Vect_Costanti : Inport  Port=4
  1-D Lookup Table : Lookup_n-D  Commented=on  NumberOfTableDimensions=1  BreakpointsForDimension1=[0,5,5.2]  Table=[42,34,0]  InternalRulePriority=Speed  RndMeth=Simplest  InputSameDT=on
  As2Ah : Gain  Commented=on  Gain=1/3600
  Bus Selector1 : BusSelector  OutputSignals=V
  Bus Selector2 : BusSelector  OutputSignals=Coef_Geometrici.Dprop
  Bus Selector3 : BusSelector  Commented=on  OutputSignals=V
  Bus Selector4 : BusSelector  Commented=on  OutputSignals=Coef_Geometrici.Dprop
  Compare To Constant : simulink/Logic and Bit Operations/Compare To Constant  relop=>=  const=150  OutDataTypeStr=boolean
  Compare To Constant1 : simulink/Logic and Bit Operations/Compare To Constant  Commented=on  relop=>=  const=150  OutDataTypeStr=boolean
  Constant : Constant  Value=2
  Constant1 : Constant  Value=4
  Constant2 : Constant  Value=3
  Constant3 : Constant  Value=5
  Constant4 : Constant  Commented=on  Value=2
  Constant5 : Constant  Commented=on  Value=4
  Constant6 : Constant  Commented=on  Value=3
  Constant7 : Constant  Commented=on  Value=5
  Display{,1..6} (7 alike) : Display
  Display{7..15} (9 alike) : Display  Commented=on
  Fcn : Fcn  Expr=u+1
  From : From  Commented=on  GotoTag=Power
  From1 : From  Commented=on  GotoTag=Power
  Gain : Gain  Gain=1/(0.8*37)
  Gain1 : Gain  Commented=on  Gain=2*pi/60
  Gain2 : Gain  Commented=on  Gain=1/Jprop
  Goto : Goto  Commented=on  GotoTag=Power
  Integrator : Integrator  Commented=on  InitialConditionSource=external
  Integrator1 : Integrator  Commented=on
  "KV_eng " : Constant  Commented=on  Value=200
  "LUT ELICA " : Subsystem
  LUT ELICA 1 : Subsystem  Commented=on
  LUT MOTORE : Gain  Gain=7400
  Math Function{,1..3} (4 alike) : Math  Operator=pow  SignedPower=on  SaturateOnIntegerOverflow=on
  Math Function{4..7} (4 alike) : Math  Commented=on  Operator=pow  SignedPower=on  SaturateOnIntegerOverflow=on
  PID Controller : pid_lib/PID Controller  Commented=on  Controller=PID  Form=Parallel  TimeDomain=Continuous-time  UseExternalTs=off  SampleTime=-1  IntegratorMethod=Forward Euler  FilterMethod=Forward Euler  ControllerParametersSource=internal  P=0.7  I=0.1  D=0  UseFilter=on  N=100  TunerSelectOption=Frequency Response Based  InitialConditionSource=internal  InitialConditionForIntegrator=0  InitialConditionForFilter=0  DifferentiatorICPrevScaledInput=0  ExternalReset=none  TrackingMode=off  Kt=1  LimitOutput=off  SatLimitsSource=internal  UpperSaturationLimit=inf  LowerSaturationLimit=-inf  LinearizeAsGain=on  AntiWindupMode=none  Kb=1  POutMin=[]  POutMax=[]  IOutMin=[]  IOutMax=[]  DOutMin=[]  DOutMax=[]  NOutMin=[]  NOutMax=[]  SumOutMin=[]  SumOutMax=[]  SaturationOutMin=[]  SaturationOutMax=[]  PParamMin=[]  PParamMax=[]  IParamMin=[]  IParamMax=[]  DParamMin=[]  DParamMax=[]  NParamMin=[]  NParamMax=[]  KbParamMin=[]  KbParamMax=[]  KtParamMin=[]  KtParamMax=[]  KbOutMin=[]  KbOutMax=[]  KtOutMin=[]  KtOutMax=[]  IntegratorOutMin=[]  IntegratorOutMax=[]  FilterOutMin=[]  FilterOutMax=[]  SumI1OutMin=[]  SumI1OutMax=[]  SumI2OutMin=[]  SumI2OutMax=[]  SumI3OutMin=[]  SumI3OutMax=[]  SumI4OutMin=[]  SumI4OutMax=[]  SumDOutMin=[]  SumDOutMax=[]  DifferentiatorOutMin=[]  DifferentiatorOutMax=[]  FilterDiffOutCoefMin=[]  FilterDiffOutCoefMax=[]  ReciprocalOutMin=[]  ReciprocalOutMax=[]  SumDenOutMin=[]  SumDenOutMax=[]  SumNumOutMin=[]  SumNumOutMax=[]  DivideOutMin=[]  DivideOutMax=[]  UdiffTsProdOutMin=[]  UdiffTsProdOutMax=[]  NTsProdOutMin=[]  NTsProdOutMax=[]  UintegralTsProdOutMin=[]  UintegralTsProdOutMax=[]  UngainTsProdOutMin=[]  UngainTsProdOutMax=[]  IntegratorContinuousStateAttributes=''  IntegratorStateMustResolveToSignalObject=off  IntegratorRTWStateStorageClass=Auto  FilterContinuousStateAttributes=''  FilterStateMustResolveToSignalObject=off  FilterRTWStateStorageClass=Auto  ParallelPVariant=InternalParameters  IdealPVariant=Disabled  IVariant=InternalParameters  DVariant=InternalParameters  IntegratorVariant=Continuous  SatVariant=Disabled  AWVariant=Passthrough  PCopyVariant=Disabled  TRVariant=Disabled  FdbkBlocksVariant=Forward  IdealPFdbkVariant=Disabled  SatFdbkVariant=Disabled  DerivativeFilterVariant=ContFilter  NVariant=InternalParameters  NCopyVariant=Disabled  FilterICVariant=InternalICsFilter  IntegratorICVariant=InternalICs  ExternalResetVariant=Disabled  TRSumVariant=Passthrough  SumFdbkVariant=Disabled  SumVariant=Sum_PID  TsampFilterVariant=InternalTs  TsampNgainVariant=Passthrough  TsampIntegralVariant=Passthrough  ExternalSaturationOutDataTypeStr=Inherit: Same as second input
  Product : Product  Commented=on  Inputs=3
  Product1 : Product  Inputs=/*/
  Product2 : Product  Inputs=****
  Product3 : Product  Inputs=****
  Product4 : Product  Commented=on  Inputs=/*/
  Product5 : Product  Commented=on  Inputs=****
  Product6 : Product  Commented=on  Inputs=****
  Product7 : Product  Commented=on  Inputs=*/
  Product8 : Product  Commented=on  Inputs=*/
  RPM->RPs : Gain  Gain=1/60
  "RPS2RPM  " : Gain  Commented=on  Gain=60
  RPs->rad/s : Gain  Gain=2*pi
  "RendimentoElica " : Gain  Commented=on  Gain=1/0.8
  "RintBatt " : Gain  Commented=on  Gain=0.013
  Saturation : Saturate  UpperLimit=1  LowerLimit=0
  Saturation1 : Saturate  Commented=on  UpperLimit=1  LowerLimit=0
  Scope : Scope
  Scope{2..6} (5 alike) : Scope  Commented=on
  Stop Simulation : Stop
  Stop Simulation1 : Stop  Commented=on
  Subsystem1 : Subsystem
  Subsystem2 : Subsystem  Commented=on
  Sum : Sum  Commented=on  Inputs=|+-
  Sum1 : Sum  Commented=on  Inputs=-+|
  Sum2 : Sum  Commented=on  Inputs=|+-
  Unit Delay : UnitDelay  InitialCondition=deltaTtrim*7400  SampleTime=-1  HasFrameUpgradeWarning=on
  Unit Delay1 : UnitDelay  Commented=on  SampleTime=0.01  HasFrameUpgradeWarning=on
  omega0eng : Constant  Commented=on  Value=439.82
  radps2RPS : Gain  Commented=on  Gain=1/(2*pi)
  "Fthrust " : Outport  VectorParamsAs1DForOutWhenUnconnected=off
  Mthrust : Outport  Port=2  VectorParamsAs1DForOutWhenUnconnected=off
  Omega : Outport  Port=3
  wires:
  Vect_Costanti/1 -> Subsystem1/4(V_cost), Bus Selector2/1
  "deltaT "/1 -> Saturation/1  "deltaT"
  V/1 -> Bus Selector1/1
  Bus Selector1/1 -> Product1/2  "<V>"
  Bus Selector2/1 -> Math Function2/1, Math Function/1, Product1/3  "<Dprop>"
  Product1/1 -> "LUT ELICA "/1(J), Display5/1
  ρ/1 -> Product2/3, Product3/2
  "LUT ELICA "/2(Cp) -> Display4/1, Product3/1
  "LUT ELICA "/1(Ct) -> Display2/1, Product2/4
  Math Function3/1 -> Product2/1
  Math Function/1 -> Product2/2
  Constant/1 -> Math Function3/2
  Constant1/1 -> Math Function/2
  Math Function2/1 -> Product3/3
  Constant3/1 -> Math Function2/2
  Constant2/1 -> Math Function1/2
  Math Function1/1 -> Product3/4
  Product2/1 -> Scope/1, Display/1, Subsystem1/1(T)
  Subsystem1/1(Fthrust) -> "Fthrust "/1
  Subsystem1/2("Mthrust ") -> Mthrust/1
  Product3/1 -> Gain/1, Display3/1, Subsystem1/2(P)
  Gain/1 -> Display6/1, Compare To Constant/1
  Compare To Constant/1 -> Stop Simulation/1
  RPs->rad/s/1 -> Omega/1
  RPM->RPs/1 -> RPs->rad/s/1, Subsystem1/3(RPS), Math Function1/1, Display1/1, Math Function3/1, Product1/1
  Saturation/1 -> LUT MOTORE/1
  Unit Delay/1 -> "LUT ELICA "/2(RPM), RPM->RPs/1
  LUT MOTORE/1 -> Fcn/1
  Fcn/1 -> Unit Delay/1
  omega0eng/1 -> Integrator/2
  Saturation1/1 -> Product/1
  Product/1 -> Gain1/1  "RPMrequ"
  From1/1 -> "RendimentoElica "/1
  Product7/1 -> Sum1/1  "disturbTorque"
  "RendimentoElica "/1 -> Product8/1
  "RintBatt "/1 -> Sum2/2  "Ah"
  Unit Delay1/1 -> "RintBatt "/1
  Sum2/1 -> Product8/2, Scope5/1, Display14/1, Product/3
  LUT ELICA 1/1(Ct) -> Display9/1, Product5/4
  Product8/1 -> Scope6/1, Compare To Constant1/1, Unit Delay1/1, Integrator1/1  "I"
  Bus Selector4/1 -> Math Function6/1, Math Function4/1, Product4/3  "<Dprop>"
  PID Controller/1 -> Sum1/2  "elecTorque"
  Integrator/1 -> Sum/2, Scope2/1, Product7/2, radps2RPS/1  "omegaeff"
  1-D Lookup Table/1 -> Display15/1, Sum2/1  "Vbatt"
  "KV_eng "/1 -> Product/2
  Math Function6/1 -> Product6/3
  Gain1/1 -> Sum/1  "radpSreq"
  Product6/1 -> Scope4/1, Display10/1, Goto/1, Subsystem2/2(P)  "Power"
  Sum1/1 -> Gain2/1  "torque"
  Compare To Constant1/1 -> Stop Simulation1/1
  LUT ELICA 1/2(Cp) -> Display11/1, Product6/1
  Integrator1/1 -> As2Ah/1  "As"
  Math Function7/1 -> Product5/1
  Sum/1 -> PID Controller/1  "error"
  As2Ah/1 -> Display13/1, 1-D Lookup Table/1  "Ah"
  Product5/1 -> Scope3/1, Display7/1, Subsystem2/1(T)
  Math Function5/1 -> Product6/4
  "RPS2RPM  "/1 -> LUT ELICA 1/2(RPM)  "RPM"
  From/1 -> Product7/1
  Math Function4/1 -> Product5/2
  Constant4/1 -> Math Function7/2
  Constant6/1 -> Math Function5/2
  Constant7/1 -> Math Function6/2
  Product4/1 -> Display12/1, LUT ELICA 1/1(J)
  radps2RPS/1 -> "RPS2RPM  "/1, Subsystem2/3(RPS), Math Function5/1, Display8/1, Math Function7/1, Product4/1  "RPS"
  Gain2/1 -> Integrator/1
  Bus Selector3/1 -> Product4/2  "<V>"
  Constant5/1 -> Math Function4/2

== system autopilota_v_22_last/Subsystem1/CONTROLLI INTERNI E SWITCH1/AENEA II_SITL1/Subsystem ==
  xE : Inport
  Φvect : Inport  Port=2
  Vb : Inport  Port=3
  ω_b : Inport  Port=4
  Bus Creator1 : BusCreator  Inputs=4
  Bus Creator{3..4,8..9} (4 alike) : BusCreator  Inputs=3
  Demux{1..2,6..7} (4 alike) : Demux  Outputs=3
  Scope : Scope
  "Xstato " : Outport  VectorParamsAs1DForOutWhenUnconnected=off
  wires:
  Demux2/3 -> Bus Creator4/3  "r"
  Bus Creator4/1 -> Bus Creator1/3  "ωvect"
  Φvect/1 -> Demux6/1
  Vb/1 -> Demux7/1
  Bus Creator8/1 -> Bus Creator1/2  "PhiThetaPsi"
  Demux1/3 -> Bus Creator3/3  "h"
  Demux2/2 -> Bus Creator4/2  "q"
  Demux2/1 -> Bus Creator4/1  "p"
  Bus Creator3/1 -> Bus Creator1/4  "xyz"
  ω_b/1 -> Demux2/1
  Demux6/3 -> Scope/1, Bus Creator8/3  "Psi"
  Demux6/1 -> Bus Creator8/1  "Phi"
  Demux1/1 -> Bus Creator3/1  "x"
  Demux7/1 -> Bus Creator9/1  "u"
  Demux7/3 -> Bus Creator9/3  "w"
  Bus Creator9/1 -> Bus Creator1/1  "uvw"
  Demux1/2 -> Bus Creator3/2  "y"
  Demux7/2 -> Bus Creator9/2  "v"
  Demux6/2 -> Bus Creator8/2  "Theta"
  Bus Creator1/1 -> "Xstato "/1  "Xstato"
  xE/1 -> Demux1/1
